simulink library "threeTetherThreeSurfaceCtrl_cl"  (R2018b)
settings: Solver=VariableStepAuto  StartTime=0.0  StopTime=10.0  RelTol=1e-3
undefined symbols (not defined in the file): ctrl
libraries: filteredPIDController_ul x6
settings Model: Creator=mcobb  LastModifiedBy=mcobb

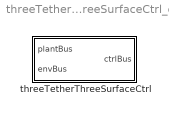
== system threeTetherThreeSurfaceCtrl_cl ==
  threeTetherThreeSurfaceCtrl : Subsystem  VariantControl=VSS_controller_threeTetherThreeSurfaceCtrl

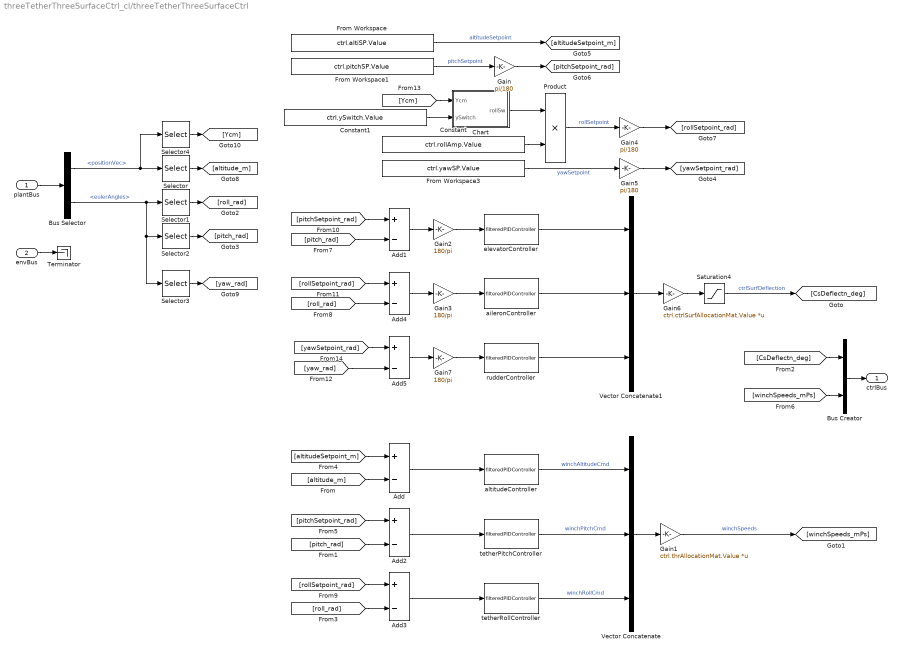
== system threeTetherThreeSurfaceCtrl_cl/threeTetherThreeSurfaceCtrl ==
  plantBus : Inport  OutDataTypeStr=Bus: plantBus
  envBus : Inport  Port=2  OutDataTypeStr=Bus: envBus
  Add{,1..5} (6 alike) : Sum  Inputs=+-
  Bus Creator : BusCreator  Inputs=2  OutDataTypeStr=Bus: fltCtrlBus
  Bus Selector : BusSelector  OutputSignals=positionVec,eulerAngles
  Chart : Stateflow chart  TreatAsAtomicUnit=on
  Constant : Constant  Value=ctrl.rollAmp.Value
  Constant1 : Constant  Value=ctrl.ySwitch.Value
  From Workspace : FromWorkspace  VariableName=ctrl.altiSP.Value  SampleTime=0
  From Workspace1 : FromWorkspace  VariableName=ctrl.pitchSP.Value  SampleTime=0
  From Workspace3 : FromWorkspace  VariableName=ctrl.yawSP.Value  SampleTime=0
  Gain : Gain  Gain=pi/180
  Gain1 : Gain  Gain=ctrl.thrAllocationMat.Value  Multiplication=Matrix(K*u)
  Gain2 : Gain  Gain=180/pi
  Gain3 : Gain  Gain=180/pi
  Gain4 : Gain  Gain=pi/180
  Gain5 : Gain  Gain=pi/180
  Gain6 : Gain  Gain=ctrl.ctrlSurfAllocationMat.Value  Multiplication=Matrix(K*u)
  Gain7 : Gain  Gain=180/pi
  Product : Product
  Saturation4 : Saturate  UpperLimit=ctrl.outputSat.upperLimit.Value  LowerLimit=ctrl.outputSat.lowerLimit.Value
  Selector : Selector  InputPortWidth=3  IndexOptions=Index vector (dialog)  Indices=3  OutputSizes=1
  Selector1 : Selector  InputPortWidth=3  IndexOptions=Index vector (dialog)  Indices=1  OutputSizes=1
  Selector2 : Selector  InputPortWidth=3  IndexOptions=Index vector (dialog)  Indices=2  OutputSizes=1
  Selector3 : Selector  InputPortWidth=3  IndexOptions=Index vector (dialog)  Indices=3  OutputSizes=1
  Selector4 : Selector  InputPortWidth=3  IndexOptions=Index vector (dialog)  Indices=2  OutputSizes=1
  Terminator : Terminator
  Vector Concatenate : Concatenate  NumInputs=3
  Vector Concatenate1 : Concatenate  NumInputs=3
  aileronController : filteredPIDController_ul/filteredPIDController  kp=ctrl.ailerons.kp.Value  ki=ctrl.ailerons.ki.Value  kd=ctrl.ailerons.kd.Value  Value=ctrl.ailerons.tau.Value
  altitudeController : filteredPIDController_ul/filteredPIDController  kp=ctrl.tetherAlti.kp.Value  ki=ctrl.tetherAlti.ki.Value  kd=ctrl.tetherAlti.kd.Value  Value=ctrl.tetherAlti.tau.Value
  elevatorController : filteredPIDController_ul/filteredPIDController  kp=ctrl.elevators.kp.Value  ki=ctrl.elevators.ki.Value  kd=ctrl.elevators.kd.Value  Value=ctrl.elevators.tau.Value
  rudderController : filteredPIDController_ul/filteredPIDController  kp=ctrl.rudder.kp.Value  ki=ctrl.rudder.ki.Value  kd=ctrl.rudder.kd.Value  Value=ctrl.rudder.tau.Value
  tetherPitchController : filteredPIDController_ul/filteredPIDController  kp=ctrl.tetherPitch.kp.Value  ki=ctrl.tetherPitch.ki.Value  kd=ctrl.tetherPitch.kd.Value  Value=ctrl.tetherPitch.tau.Value
  tetherRollController : filteredPIDController_ul/filteredPIDController  kp=ctrl.tetherRoll.kp.Value  ki=ctrl.tetherRoll.ki.Value  kd=ctrl.tetherRoll.kd.Value  Value=ctrl.tetherRoll.tau.Value
  ctrlBus : Outport  OutDataTypeStr=Bus: fltCtrlBus
  wires:
  Vector Concatenate/1 -> Gain1/1
  Add2/1 -> tetherPitchController/1
  Add3/1 -> tetherRollController/1
  Add/1 -> altitudeController/1
  [pitchSetpoint_rad] -> Add2/1
  [pitch_rad] -> Add2/2
  [roll_rad] -> Add3/2
  [rollSetpoint_rad] -> Add3/1
  tetherRollController/1 -> Vector Concatenate/3  "winchRollCmd"
  [altitude_m] -> Add/2
  [altitudeSetpoint_m] -> Add/1
  tetherPitchController/1 -> Vector Concatenate/2  "winchPitchCmd"
  altitudeController/1 -> Vector Concatenate/1  "winchAltitudeCmd"
  Saturation4/1 -> [CsDeflectn_deg]  "ctrlSurfDeflection"
  Vector Concatenate1/1 -> Gain6/1
  aileronController/1 -> Vector Concatenate1/2
  elevatorController/1 -> Vector Concatenate1/1
  [roll_rad] -> Add4/2
  Add4/1 -> Gain3/1
  [pitch_rad] -> Add1/2
  Gain6/1 -> Saturation4/1
  Gain2/1 -> elevatorController/1
  Gain3/1 -> aileronController/1
  Add1/1 -> Gain2/1
  Bus Creator/1 -> ctrlBus/1
  Gain1/1 -> [winchSpeeds_mPs]  "winchSpeeds"
  [CsDeflectn_deg] -> Bus Creator/1
  [winchSpeeds_mPs] -> Bus Creator/2
  envBus/1 -> Terminator/1
  plantBus/1 -> Bus Selector/1
  Gain/1 -> [pitchSetpoint_rad]
  Gain4/1 -> [rollSetpoint_rad]
  Selector/1 -> [altitude_m]
  [pitchSetpoint_rad] -> Add1/1
  [rollSetpoint_rad] -> Add4/1
  Bus Selector/1 -> Selector4/1, Selector/1  "<positionVec>"
  Bus Selector/2 -> Selector3/1, Selector2/1, Selector1/1  "<eulerAngles>"
  Selector1/1 -> [roll_rad]
  Selector2/1 -> [pitch_rad]
  From Workspace/1 -> [altitudeSetpoint_m]  "altitudeSetpoint"
  From Workspace1/1 -> Gain/1  "pitchSetpoint"
  Product/1 -> Gain4/1  "rollSetpoint"
  From Workspace3/1 -> Gain5/1  "yawSetpoint"
  Gain5/1 -> [yawSetpoint_rad]
  [yaw_rad] -> Add5/2
  Add5/1 -> Gain7/1
  [yawSetpoint_rad] -> Add5/1
  Gain7/1 -> rudderController/1
  rudderController/1 -> Vector Concatenate1/3
  Selector3/1 -> [yaw_rad]
  Selector4/1 -> [Ycm]
  [Ycm] -> Chart/1(Ycm)
  Constant/1 -> Product/2
  Chart/1(rollSw) -> Product/1
  Constant1/1 -> Chart/2(ySwitch)

== stateflow chart threeTetherThreeSurfaceCtrl_cl/threeTetherThreeSurfaceCtrl/Chart ==
  state PositiveRoll
    entry:
    rollSw = 1;
  state NegativeRoll
    entry:
    rollSw = -1;
  (default) -> PositiveRoll
  NegativeRoll -> PositiveRoll : [Ycm>ySwitch]
  PositiveRoll -> NegativeRoll : [Ycm<-ySwitch]
  data: Ycm input; rollSw output; ySwitch input
